simulink library "determineIterationPhase_ul"  (R2018a)
settings: Solver=VariableStepAuto  StartTime=0.0  StopTime=10.0  RelTol=1e-3
undefined symbols (not defined in the file or in its folder): ctrl, iterationPhase_enum
libraries: simulink x2
settings Model: Creator=mitch  LastModifiedBy=mitch

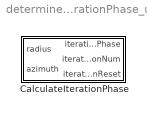
== system determineIterationPhase_ul ==
  CalculateIterationPhase : Subsystem

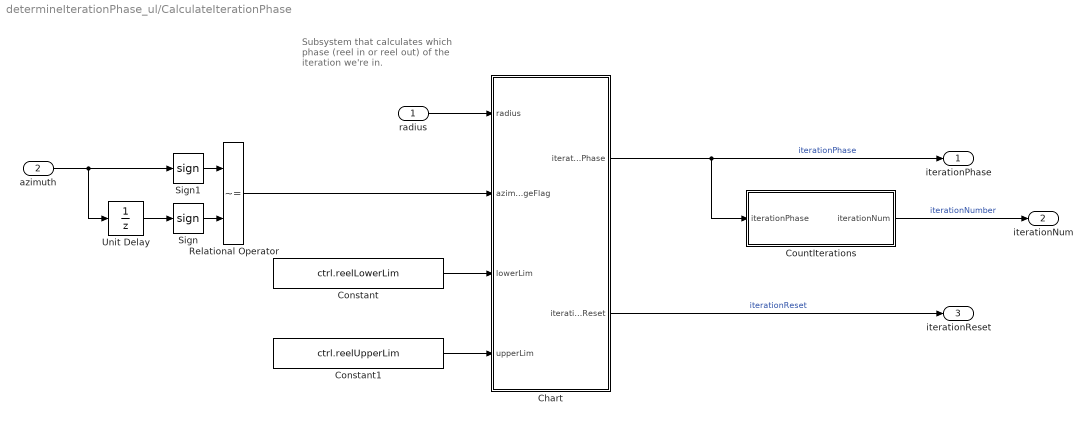
== system determineIterationPhase_ul/CalculateIterationPhase ==
  note: Subsystem that calculates which
      | phase (reel in or reel out) of the
      | iteration we're in.
  radius : Inport
  azimuth : Inport  Port=2
  Chart : Stateflow chart  TreatAsAtomicUnit=on
  Constant : Constant  Value=ctrl.reelLowerLim
  Constant1 : Constant  Value=ctrl.reelUpperLim
  CountIterations : Subsystem
  Relational Operator : RelationalOperator  Operator=~=  OutDataTypeStr=boolean  RndMeth=Simplest
  Sign : Signum
  Sign1 : Signum
  Unit Delay : UnitDelay  SampleTime=-1
  iterationPhase : Outport  OutDataTypeStr=Enum: iterationPhase_enum
  iterationNum : Outport  Port=2  OutDataTypeStr=uint32
  iterationReset : Outport  Port=3  OutDataTypeStr=boolean
  wires:
  Chart/2(iterationReset) -> iterationReset/1  "iterationReset"
  radius/1 -> Chart/1(radius)
  Relational Operator/1 -> Chart/2(azimuthSignChangeFlag)
  Sign/1 -> Relational Operator/2
  Sign1/1 -> Relational Operator/1
  azimuth/1 -> Unit Delay/1, Sign1/1
  Unit Delay/1 -> Sign/1
  Constant/1 -> Chart/3(lowerLim)
  Constant1/1 -> Chart/4(upperLim)
  Chart/1(iterationPhase) -> CountIterations/1(iterationPhase), iterationPhase/1  "iterationPhase"
  CountIterations/1(iterationNum) -> iterationNum/1  "iterationNumber"

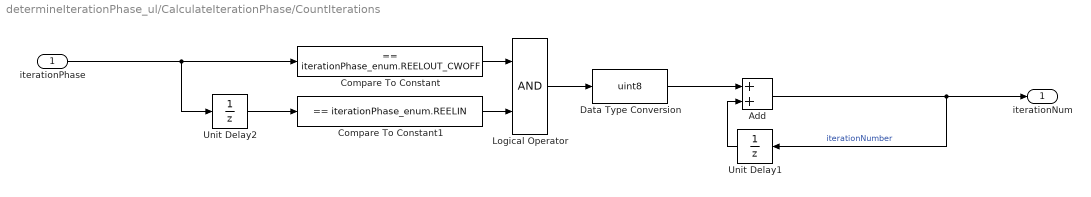
== system determineIterationPhase_ul/CalculateIterationPhase/CountIterations ==
  iterationPhase : Inport
  Add : Sum
  Compare To Constant : simulink/Logic and Bit Operations/Compare To Constant  relop===  const=iterationPhase_enum.REELOUT_CWOFF  OutDataTypeStr=boolean
  Compare To Constant1 : simulink/Logic and Bit Operations/Compare To Constant  relop===  const=iterationPhase_enum.REELIN  OutDataTypeStr=boolean
  Data Type Conversion : DataTypeConversion  OutDataTypeStr=uint8
  Logical Operator : Logic  AllPortsSameDT=off  OutDataTypeStr=boolean
  Unit Delay1 : UnitDelay  InitialCondition=1  SampleTime=-1
  Unit Delay2 : UnitDelay  InitialCondition=iterationPhase_enum.REELOUT_CWOFF  SampleTime=-1
  iterationNum : Outport
  wires:
  Logical Operator/1 -> Data Type Conversion/1
  Unit Delay1/1 -> Add/2
  Add/1 -> iterationNum/1, Unit Delay1/1  "iterationNumber"
  Compare To Constant1/1 -> Logical Operator/2
  Unit Delay2/1 -> Compare To Constant1/1
  iterationPhase/1 -> Unit Delay2/1, Compare To Constant/1
  Compare To Constant/1 -> Logical Operator/1
  Data Type Conversion/1 -> Add/1

== stateflow chart determineIterationPhase_ul/CalculateIterationPhase/Chart ==
  state REELOUT_CWON
    state NORMAL
      entry: iterationReset = false;
    state RESET
      entry: iterationReset = true;
    (default) -> NORMAL
    RESET -> NORMAL : after(1,tick)
  state REELOUT_CWOFF
  state REELIN
  REELOUT_CWOFF -> RESET : [radius>lowerLim]
  (default) -> (junction 18)
  (junction 18) -> REELOUT_CWON [order 1] : [radius<=upperLim]
  (junction 18) -> (junction 17) [order 2]
  REELOUT_CWON -> REELIN : [radius>upperLim && ...
      | azimuthSignChangeFlag]
  REELIN -> REELOUT_CWOFF : [radius<lowerLim]
  (junction 17) -> REELIN
  data: radius input double; azimuthSignChangeFlag input boolean; iterationPhase output Enum: iterationPhase_enum; lowerLim input double; upperLim input double; iterationReset output boolean
